simulink model "wrench_observer_R2016b"  (R2016b)
settings: Solver=VariableStepAuto  StartTime=0.0  StopTime=0.75  RelTol=1e-3
InitFcn:
  | %x_k1 = 0.00001*ones(36,1); % initialisation with initial state uncertainity
  | %P_k1 = 0.00001*ones(36); % initialisation with initial state uncertainity
values from neighbouring files (symbols this model uses):
  a_noise = 0    [parameter.m]
  alpha1 = pi/2    (= 1.57079632679)    [parameter.m]
  alpha2 = 0    [parameter.m]
  alpha3 = 0    [parameter.m]
  angular_noise = 0    [parameter.m]
  g = 9.81    [parameter.m]
  K_f_comm = 1    [parameter.m]
  K_I = [500*eye(3), zeros(3), zeros(3) ... (first row only)    [parameter.m]
  K_tau_comm = 1    [parameter.m]
  K_tau_man_comm = 1    [parameter.m]
  m = 3.9    [parameter.m]
  m_l1 = 0.3    [parameter.m]
  m_l2 = 0.35    [parameter.m]
  m_l3 = 0.35    [parameter.m]
  N_m = 1*diag([(p_noise/(3*noise_factor))^2 (p_noise/(3*noise_factor))^2 (p_noise/(3*noise_factor))^2 (a_noise/(3*noise_factor))^2 (a_noise/(3*noise_factor))^2 (a_noise/(3*noise_factor))^2 (angular_noise/(3*noise_factor))^2 (angular_noise/(3*noise_factor))^2 (angular_noise/(3*noise_factor))^2 (omega_noise/(3*noise_factor))^2 (omega_noise/(3*noise_factor))^2 (omega_noise/(3*noise_factor))^2 (theta_noise/( ...(+272 chars)    [parameter.m]
  N_p = diag(noise_factor_EKF)    [parameter.m]
  omega_dot_noise = 0    [parameter.m]
  omega_noise = 0    [parameter.m]
  p_L1_l1 = [p_L1_x_l1 p_L1_y_l1 p_L1_z_l1]'    [parameter.m]
  p_L2_l2 = [p_L2_x_l2 p_L2_y_l2 p_L2_z_l2]'    [parameter.m]
  p_L3_l3 = [p_L3_x_l3 p_L3_y_l3 p_L3_z_l3]'    [parameter.m]
  p_noise = 0    [parameter.m]
  R_B_L0 = [1 0 0;0 1 0; 0 0 1]    [parameter.m]
  T_delay = 0    [parameter.m]
  T_dis = 0.01    [parameter.m]
  theta_dot_dot_noise = 0    [parameter.m]
  theta_dot_noise = 0    [parameter.m]
  theta_noise = 0    [parameter.m]
  Ts = 1/250    (= 0.004)    [parameter.m]
  v_noise = 0    [parameter.m]
libraries: simulink x9, dspstat3 x2, dspinverses x1
(part 4 of 5)

== matlab function wrench_observer_R2016b/Subsystem/MATLAB Function ==
  data: theta input; J_transpose output
function J_transpose = fcn(theta)
theta1 = theta(1);
theta2 = theta(2);
theta3 = theta(3);
% J = [ -cos(theta1)*((3*sin(theta2 + theta3))/10 + (3*sin(theta2))/10), -(3*sin(theta2 + theta3)*cos(theta1))/10,0;
% -sin(theta1)*((3*sin(theta2 + theta3))/10 + (3*sin(theta2))/10), -(3*sin(theta2 + theta3)*sin(theta1))/10,0;
% (3*cos(theta2 + theta3))/10 + (3*cos(theta2))/10,(3*cos(theta2 + theta3))/10,0;
% sin(theta1),sin(theta1),sin(theta1);
% -cos(theta1), -cos(theta1), -cos(theta1);
% 0,0,0];
J = [ -(3*cos(theta2 + theta3)*sin(theta1))/10, -cos(theta1)*((3*sin(theta2 + theta3))/10 - 1/10), -(3*cos(theta1)*(sin(theta2 + theta3) - sin(theta2)))/10;
      (3*cos(theta2 + theta3)*cos(theta1))/10, -sin(theta1)*((3*sin(theta2 + theta3))/10 - 1/10), -(3*sin(theta1)*(sin(theta2 + theta3) - sin(theta2)))/10;
      0, (3*cos(theta2 + theta3))/10, (3*cos(theta2 + theta3))/10 - (3*cos(theta2))/10;
      0, sin(theta1),sin(theta1);
      0,-cos(theta1), -cos(theta1);
      1, 0,0];

J_transpose = J';

== matlab function wrench_observer_R2016b/Wrench Observer EKF/MATLAB Function3 ==
  data: C output
function C = fcn()
C = [ 	1, 	0, 	0, 	0, 	0, 	0, 	0, 	0, 	0, 	0, 	0, 	0, 	0, 	0, 	0, 	0, 	0, 	0, 	0, 	0, 	0, 	0, 	0, 	0, 	0, 	0, 	0, 	0, 	0, 	0, 	0, 	0, 	0, 	0, 	0, 	0; 
		0, 	1, 	0, 	0, 	0, 	0, 	0, 	0, 	0, 	0, 	0, 	0, 	0, 	0, 	0, 	0, 	0, 	0, 	0, 	0, 	0, 	0, 	0, 	0, 	0, 	0, 	0, 	0, 	0, 	0, 	0, 	0, 	0, 	0, 	0, 	0; 
		0, 	0, 	1, 	0, 	0, 	0, 	0, 	0, 	0, 	0, 	0, 	0, 	0, 	0, 	0, 	0, 	0, 	0, 	0, 	0, 	0, 	0, 	0, 	0, 	0, 	0, 	0, 	0, 	0, 	0, 	0, 	0, 	0, 	0, 	0, 	0; 
		0, 	0, 	0, 	0, 	0, 	0, 	3783/392000000000 - (3^(1/2)*((3*3^(1/2))/20 - 1/10))/9800000 - (3*3^(1/2))/7000000000, 	- (9*3^(1/2))/28000000000 - (3^(1/2)*((3*3^(1/2))/20 - 1/10))/9800000 - 52641/784000000000, 	- (3*3^(1/2))/28000000000 - (3^(1/2)*((3*3^(1/2))/20 - 1/10))/4900000 - 53013/784000000000, 	- (3*3^(1/2))/2800000 - 3/9800000, 	381/7840000, 	- (3*3^(1/2))/2800000 - (3^(1/2)*((3*3^(1/2))/20 - 1/10))/1960 - 237/156800000, 	(35937*3^(1/2))/7840000000000 + 1/490000000, 	(35397*3^(1/2))/7840000000000 + 9/28000000000, 	(177*3^(1/2))/392000000000 + 3/17500000000, 	- (3*3^(1/2)*((3*3^(1/2))/20 - 1/10))/1960 - 27/196000, 	-687/1600000, 	-23643/156800000, 	10/49, 	0, 	0, 	10/49, 	0, 	0, 	0, 	0, 	0, 	0, 	0, 	0, 	0, 	0, 	0, 	0, 	0, 	0; 
		0, 	0, 	0, 	0, 	0, 	0, 	- (243969*3^(1/2))/3920000000000 - 26389/245000000000, 	(26073*3^(1/2))/1960000000000 - 991/61250000000, 	- (179727*3^(1/2))/3920000000000 - 110003/980000000000, 	-381/784000, 	- (303*3^(1/2))/56000000 - 303/196000000, 	(56073*3^(1/2))/784000000 - 10303/196000000, 	- (3^(1/2)*((3*3^(1/2))/20 - 1/10))/49000000 - 60189/7840000000000, 	(249*3^(1/2))/392000000000 - 192873/7840000000000, 	- (3561*3^(1/2))/784000000000 - 990219/39200000000000, 	(3*3^(1/2))/39200 - 3/9800, 	- (35979*3^(1/2))/78400000 - 3/9800, 	- (23979*3^(1/2))/156800000 - 3/112000, 	0, 	10/49, 	0, 	0, 	10/49, 	0, 	0, 	0, 	0, 	0, 	0, 	0, 	0, 	0, 	0, 	0, 	0, 	0; 
		0, 	0, 	0, 	0, 	0, 	0, 	(39969*3^(1/2))/392000000000 + (3^(1/2)*((3*3^(1/2))/20 - 1/10))/9800000 + 5337/196000000000, 	(3^(1/2)*((3*3^(1/2))/20 - 1/10))/9800000 - (24273*3^(1/2))/392000000000 + 1429/14000000000, 	(561*3^(1/2))/56000000000 + 5331/196000000000, 	(3*3^(1/2))/28000 + (3^(1/2)*((3*3^(1/2))/20 - 1/10))/1960 + 237/1568000, 	5003/9800000 - (60231*3^(1/2))/78400000, 	0, 	(183*3^(1/2))/78400000000 + (3^(1/2)*((3*3^(1/2))/20 - 1/10))/9800000 - 611/784000000000, 	24147/784000000000 - (14871*3^(1/2))/3920000000000, 	17601/980000000000 - (24021*3^(1/2))/7840000000000, 	(3^(1/2)*((3*3^(1/2))/20 - 1/10))/1960 - (9*3^(1/2))/19600 + 1/1960, 	(2379*3^(1/2))/7840000 + 9/112000, 	(4779*3^(1/2))/15680000 + 9/224000, 	0, 	0, 	10/49, 	0, 	0, 	10/49, 	0, 	0, 	0, 	0, 	0, 	0, 	0, 	0, 	0, 	0, 	0, 	0; 
		0, 	0, 	0, 	0, 	0, 	0, 	1, 	0, 	0, 	0, 	0, 	0, 	0, 	0, 	0, 	0, 	0, 	0, 	0, 	0, 	0, 	0, 	0, 	0, 	0, 	0, 	0, 	0, 	0, 	0, 	0, 	0, 	0, 	0, 	0, 	0; 
		0, 	0, 	0, 	0, 	0, 	0, 	0, 	1, 	0, 	0, 	0, 	0, 	0, 	0, 	0, 	0, 	0, 	0, 	0, 	0, 	0, 	0, 	0, 	0, 	0, 	0, 	0, 	0, 	0, 	0, 	0, 	0, 	0, 	0, 	0, 	0; 
		0, 	0, 	0, 	0, 	0, 	0, 	0, 	0, 	1, 	0, 	0, 	0, 	0, 	0, 	0, 	0, 	0, 	0, 	0, 	0, 	0, 	0, 	0, 	0, 	0, 	0, 	0, 	0, 	0, 	0, 	0, 	0, 	0, 	0, 	0, 	0; 
		0, 	0, 	0, 	0, 	0, 	0, 	0, 	0, 	0, 	1, 	0, 	0, 	0, 	0, 	0, 	0, 	0, 	0, 	0, 	0, 	0, 	0, 	0, 	0, 	0, 	0, 	0, 	0, 	0, 	0, 	0, 	0, 	0, 	0, 	0, 	0; 
		0, 	0, 	0, 	0, 	0, 	0, 	0, 	0, 	0, 	0, 	1, 	0, 	0, 	0, 	0, 	0, 	0, 	0, 	0, 	0, 	0, 	0, 	0, 	0, 	0, 	0, 	0, 	0, 	0, 	0, 	0, 	0, 	0, 	0, 	0, 	0; 
		0, 	0, 	0, 	0, 	0, 	0, 	0, 	0, 	0, 	0, 	0, 	1, 	0, 	0, 	0, 	0, 	0, 	0, 	0, 	0, 	0, 	0, 	0, 	0, 	0, 	0, 	0, 	0, 	0, 	0, 	0, 	0, 	0, 	0, 	0, 	0; 
		0, 	0, 	0, 	0, 	0, 	0, 	0, 	0, 	0, 	0, 	0, 	0, 	1, 	0, 	0, 	0, 	0, 	0, 	0, 	0, 	0, 	0, 	0, 	0, 	0, 	0, 	0, 	0, 	0, 	0, 	0, 	0, 	0, 	0, 	0, 	0; 
		0, 	0, 	0, 	0, 	0, 	0, 	0, 	0, 	0, 	0, 	0, 	0, 	0, 	1, 	0, 	0, 	0, 	0, 	0, 	0, 	0, 	0, 	0, 	0, 	0, 	0, 	0, 	0, 	0, 	0, 	0, 	0, 	0, 	0, 	0, 	0; 
		0, 	0, 	0, 	0, 	0, 	0, 	0, 	0, 	0, 	0, 	0, 	0, 	0, 	0, 	1, 	0, 	0, 	0, 	0, 	0, 	0, 	0, 	0, 	0, 	0, 	0, 	0, 	0, 	0, 	0, 	0, 	0, 	0, 	0, 	0, 	0; 
		0, 	0, 	0, 	((3^(1/2)*((3*3^(1/2))/20 - 1/10))/400 + 27/40000)/(100*((3*3^(1/2))/100000000 - 31/400000000)) + 28569/(6400000000*((3*3^(1/2))/100000000 - 31/400000000)), 	((3*3^(1/2))/8000 + 1/1000)/(100*((3*3^(1/2))/100000000 - 31/400000000)) - ((21*3^(1/2))/16000000 + 3/2000)/(200*((3*3^(1/2))/100000000 - 31/400000000)) + ((23979*3^(1/2))/32000000 + 21/160000)/(200*((3*3^(1/2))/100000000 - 31/400000000)), 	((21*3^(1/2))/1600000 - 63/160000)/(200*((3*3^(1/2))/100000000 - 31/400000000)) - ((4779*3^(1/2))/3200000 + 63/320000)/(200*((3*3^(1/2))/100000000 - 31/400000000)) - ((3^(1/2)*((3*3^(1/2))/20 - 1/10))/400 - (9*3^(1/2))/4000 + 1/400)/(100*((3*3^(1/2))/100000000 - 31/400000000)), 	((5121*3^(1/2)*((3*3^(1/2))/20 - 1/10))/40000000000000 - (4876773983*3^(1/2))/32000000000000000 + 111056949/800000000000000)/(100*((3*3^(1/2))/100000000 - 31/400000000)) - ((9397082859*3^(1/2))/64000000000000000 + (21*3^(1/2)*((3*3^(1/2))/20 - 1/10))/160000000000 + 346647/20000000000000)/(200*((3*3^(1/2))/100000000 - 31/400000000)) - ((1183480443*3^(1/2))/80000000000000000 + (21*3^(1/2)*((3*3^(1/2))/20 - 1/10))/3200000000000 - 16010785891/800000000000000)/(10*((3*3^(1/2))/100000000 - 31/400000000)) + ((1665944541*3^(1/2))/32000000000000000 + (3831*3^(1/2)*((3*3^(1/2))/20 - 1/10))/200000000000000 - 160128933757/8000000000000000)/(5*((3*3^(1/2))/100000000 - 31/400000000)) + ((377787*3^(1/2))/200000000000000 - 27893859/80000000000000)/(200*((3*3^(1/2))/100000000 - 31/400000000)) + ((5185251*3^(1/2))/16000000000000000 + 31944083711/1600000000000000)/(10*((3*3^(1/2))/100000000 - 31/400000000)) - (((21*3^(1/2))/20000000 - 217/80000000)*((5185251*3^(1/2))/16000000000000000 + 31944083711/1600000000000000))/(200*((3*3^(1/2))/100000000 - 31/400000000)^2) + (((21*3^(1/2))/20000000 - 217/80000000)*((1183480443*3^(1/2))/80000000000000000 + (21*3^(1/2)*((3*3^(1/2))/20 - 1/10))/3200000000000 - 16010785891/800000000000000))/(200*((3*3^(1/2))/100000000 - 31/400000000)^2) - (((21*3^(1/2))/20000000 - 217/80000000)*((1665944541*3^(1/2))/32000000000000000 + (3831*3^(1/2)*((3*3^(1/2))/20 - 1/10))/200000000000000 - 160128933757/8000000000000000))/(100*((3*3^(1/2))/100000000 - 31/400000000)^2), 	((1665944541*3^(1/2))/32000000000000000 + (3831*3^(1/2)*((3*3^(1/2))/20 - 1/10))/200000000000000 - 160128933757/8000000000000000)/(5*((3*3^(1/2))/100000000 - 31/400000000)) - ((3795389037*3^(1/2))/12800000000000000 + (21*3^(1/2)*((3*3^(1/2))/20 - 1/10))/320000000000 - 27840879/160000000000000)/(200*((3*3^(1/2))/100000000 - 31/400000000)) - ((1183480443*3^(1/2))/80000000000000000 + (21*3^(1/2)*((3*3^(1/2))/20 - 1/10))/3200000000000 - 16010785891/800000000000000)/(10*((3*3^(1/2))/100000000 - 31/400000000)) - ((2482807*3^(1/2)*((3*3^(1/2))/20 - 1/10))/5000000000000 - (11772968963*3^(1/2))/32000000000000000 + 61404471/200000000000000)/(100*((3*3^(1/2))/100000000 - 31/400000000)) + ((3210399*3^(1/2))/800000000000000 - (3*3^(1/2)*((3*3^(1/2))/20 - 1/10))/2000000000 + 4331121/160000000000000)/(200*((3*3^(1/2))/100000000 - 31/400000000)) + ((5185251*3^(1/2))/16000000000000000 + 31944083711/1600000000000000)/(10*((3*3^(1/2))/100000000 - 31/400000000)) + (((3*3^(1/2))/4000000 - 31/16000000)*((1183480443*3^(1/2))/80000000000000000 + (21*3^(1/2)*((3*3^(1/2))/20 - 1/10))/3200000000000 - 16010785891/800000000000000))/(200*((3*3^(1/2))/100000000 - 31/400000000)^2) - (((3*3^(1/2))/4000000 - 31/16000000)*((1665944541*3^(1/2))/32000000000000000 + (3831*3^(1/2)*((3*3^(1/2))/20 - 1/10))/200000000000000 - 160128933757/8000000000000000))/(100*((3*3^(1/2))/100000000 - 31/400000000)^2) - (((3*3^(1/2))/4000000 - 31/16000000)*((5185251*3^(1/2))/16000000000000000 + 31944083711/1600000000000000))/(200*((3*3^(1/2))/100000000 - 31/400000000)^2), 	((114343521*3^(1/2))/1600000000000000 + (9943777*3^(1/2)*((3*3^(1/2))/20 - 1/10))/20000000000000 + 268316551/800000000000000)/(100*((3*3^(1/2))/100000000 - 31/400000000)) + ((3465639*3^(1/2))/1600000000000000 + (3*3^(1/2)*((3*3^(1/2))/20 - 1/10))/2000000000 - 55575441/160000000000000)/(200*((3*3^(1/2))/100000000 - 31/400000000)) + ((2404758213*3^(1/2))/16000000000000000 - (21*3^(1/2)*((3*3^(1/2))/20 - 1/10))/320000000000 + 7131903/64000000000000)/(200*((3*3^(1/2))/100000000 - 31/400000000)) + (((3*3^(1/2))/5000000 - 31/20000000)*((1183480443*3^(1/2))/80000000000000000 + (21*3^(1/2)*((3*3^(1/2))/20 - 1/10))/3200000000000 - 16010785891/800000000000000))/(200*((3*3^(1/2))/100000000 - 31/400000000)^2) - (((3*3^(1/2))/5000000 - 31/20000000)*((1665944541*3^(1/2))/32000000000000000 + (3831*3^(1/2)*((3*3^(1/2))/20 - 1/10))/200000000000000 - 160128933757/8000000000000000))/(100*((3*3^(1/2))/100000000 - 31/400000000)^2) - (((3*3^(1/2))/5000000 - 31/20000000)*((5185251*3^(1/2))/16000000000000000 + 31944083711/1600000000000000))/(200*((3*3^(1/2))/100000000 - 31/400000000)^2), 	- ((62493*3^(1/2))/16000000000 + (249937*3^(1/2)*((3*3^(1/2))/20 - 1/10))/100000000 - 23974611/32000000000)/(100*((3*3^(1/2))/100000000 - 31/400000000)) - 60604689/(6400000000000*((3*3^(1/2))/100000000 - 31/400000000)) - ((207*3^(1/2))/1280000000 + (21*3^(1/2)*((3*3^(1/2))/20 - 1/10))/32000000 + 2114643/32000000000)/(200*((3*3^(1/2))/100000000 - 31/400000000)), 	((2107047*3^(1/2))/320000000000 - 168129/12800000000)/(200*((3*3^(1/2))/100000000 - 31/400000000)) + ((7765251*3^(1/2))/320000000000 + 5703/40000000)/(200*((3*3^(1/2))/100000000 - 31/400000000)) - ((3*3^(1/2)*((3*3^(1/2))/20 - 1/10))/8000000000 - (596441019*3^(1/2))/160000000000 + 204842381/80000000000)/(100*((3*3^(1/2))/100000000 - 31/400000000)), 	((20010287*3^(1/2)*((3*3^(1/2))/20 - 1/10))/8000000000 - (119986137*3^(1/2))/320000000000 + 40005943/160000000000)/(100*((3*3^(1/2))/100000000 - 31/400000000)) - ((1031871*3^(1/2))/1600000000000 - 121359/64000000000)/(200*((3*3^(1/2))/100000000 - 31/400000000)) - ((416349*3^(1/2))/320000000000 - 123711/32000000000)/(200*((3*3^(1/2))/100000000 - 31/400000000)), 	- ((4034511*3^(1/2))/1600000000000000 + (297*3^(1/2)*((3*3^(1/2))/20 - 1/10))/400000000000 + 16684749/16000000000000000)/(200*((3*3^(1/2))/100000000 - 31/400000000)) - ((7589019*3^(1/2))/500000000000000 + (179409213*3^(1/2)*((3*3^(1/2))/20 - 1/10))/400000000000000 - 125998557/8000000000000000)/(100*((3*3^(1/2))/100000000 - 31/400000000)) - ((52161039*3^(1/2))/3200000000000000 + (21*3^(1/2)*((3*3^(1/2))/20 - 1/10))/32000000000000 - 117174411/8000000000000000)/(200*((3*3^(1/2))/100000000 - 31/400000000)), 	((1183480443*3^(1/2))/80000000000000000 + (21*3^(1/2)*((3*3^(1/2))/20 - 1/10))/3200000000000 - 16010785891/800000000000000)/(300*((3*3^(1/2))/100000000 - 31/400000000)) + ((78898791*3^(1/2))/4000000000000000 + (21*3^(1/2)*((3*3^(1/2))/20 - 1/10))/16000000000000 + 2373464247/20000000000000000)/(200*((3*3^(1/2))/100000000 - 31/400000000)) + ((29906877*3^(1/2))/1600000000000000 + (21*3^(1/2)*((3*3^(1/2))/20 - 1/10))/32000000000000 + 5990219349/80000000000000000)/(200*((3*3^(1/2))/100000000 - 31/400000000)) + ((5185251*3^(1/2))/16000000000000000 + 31944083711/1600000000000000)/(300*((3*3^(1/2))/100000000 - 31/400000000)) - ((23697*3^(1/2)*((3*3^(1/2))/20 - 1/10))/32000000000000 - (369986349*3^(1/2))/8000000000000000 + 51614439/8000000000000000)/(100*((3*3^(1/2))/100000000 - 31/400000000)), 	((599887743*3^(1/2))/16000000000000000 - (1779879*3^(1/2)*((3*3^(1/2))/20 - 1/10))/1600000000000000 + 14540151/32000000000000000)/(100*((3*3^(1/2))/100000000 - 31/400000000)) + ((11901*3^(1/2)*((3*3^(1/2))/20 - 1/10))/32000000000000 - (4750881*3^(1/2))/2000000000000000 + 4731132549/80000000000000000)/(200*((3*3^(1/2))/100000000 - 31/400000000)) + ((29900577*3^(1/2))/1600000000000000 + (21*3^(1/2)*((3*3^(1/2))/20 - 1/10))/32000000000000 + 5997450849/80000000000000000)/(200*((3*3^(1/2))/100000000 - 31/400000000)) + (((11*3^(1/2))/200000000 - 3/40000000)*((5185251*3^(1/2))/16000000000000000 + 31944083711/1600000000000000))/(200*((3*3^(1/2))/100000000 - 31/400000000)^2) - (100*((3*3^(1/2))/20000 - 1/20000)*((1183480443*3^(1/2))/80000000000000000 + (21*3^(1/2)*((3*3^(1/2))/20 - 1/10))/3200000000000 - 16010785891/800000000000000))/(3*((3*3^(1/2))/100000000 - 31/400000000)) - (((11*3^(1/2))/200000000 - 3/40000000)*((1183480443*3^(1/2))/80000000000000000 + (21*3^(1/2)*((3*3^(1/2))/20 - 1/10))/3200000000000 - 16010785891/800000000000000))/(200*((3*3^(1/2))/100000000 - 31/400000000)^2) + (((11*3^(1/2))/200000000 - 3/40000000)*((1665944541*3^(1/2))/32000000000000000 + (3831*3^(1/2)*((3*3^(1/2))/20 - 1/10))/200000000000000 - 160128933757/8000000000000000))/(100*((3*3^(1/2))/100000000 - 31/400000000)^2) + (3^(1/2)*((1665944541*3^(1/2))/32000000000000000 + (3831*3^(1/2)*((3*3^(1/2))/20 - 1/10))/200000000000000 - 160128933757/8000000000000000))/(100*((3*3^(1/2))/100000000 - 31/400000000)) + (100*((3*3^(1/2))/20000 + 1/20000)*((5185251*3^(1/2))/16000000000000000 + 31944083711/1600000000000000))/(3*((3*3^(1/2))/100000000 - 31/400000000)), 	- ((891*3^(1/2))/80000000 - 417/40000000)/(100*((3*3^(1/2))/100000000 - 31/400000000)) - ((1192731*3^(1/2))/3200000000 - 1205067/3200000000)/(200*((3*3^(1/2))/100000000 - 31/400000000)) - ((292941*3^(1/2))/800000000 - 589209/1600000000)/(200*((3*3^(1/2))/100000000 - 31/400000000)), 	- (9*3^(1/2))/(400000000*((3*3^(1/2))/100000000 - 31/400000000)) - ((58929*3^(1/2))/160000000 - 601209/1600000000)/(200*((3*3^(1/2))/100000000 - 31/400000000)) - ((307161*3^(1/2))/800000000 - 620169/1600000000)/(100*((3*3^(1/2))/100000000 - 31/400000000)), 	((58929*3^(1/2))/160000000 - 601209/1600000000)/(200*((3*3^(1/2))/100000000 - 31/400000000)) - ((1192731*3^(1/2))/3200000000 - 1205067/3200000000)/(100*((3*3^(1/2))/100000000 - 31/400000000)), 	0, 	0, 	0, 	0, 	0, 	0, 	0, 	0, 	0, 	0, 	0, 	0, 	-1/(100*((3*3^(1/2))/100000000 - 31/400000000)), 	1/(200*((3*3^(1/2))/100000000 - 31/400000000)), 	1/(200*((3*3^(1/2))/100000000 - 31/400000000)), 	-1/(100*((3*3^(1/2))/100000000 - 31/400000000)), 	1/(200*((3*3^(1/2))/100000000 - 31/400000000)), 	1/(200*((3*3^(1/2))/100000000 - 31/400000000)); 
		0, 	0, 	0, 	(821*((3*3^(1/2))/10000 - 1/1000))/(480000*((3*3^(1/2))/100000000 - 31/400000000)) - (2627*((3*3^(1/2))/10000 - 11/20000))/(320000*((3*3^(1/2))/100000000 - 31/400000000)) - ((3^(1/2)*((3*3^(1/2))/20 - 1/10))/400 + 27/40000)/(200*((3*3^(1/2))/100000000 - 31/400000000)), 	- ((3*3^(1/2))/8000 + 1/1000)/(200*((3*3^(1/2))/100000000 - 31/400000000)) - (100*((3*3^(1/2))/10000 - 1/1000)*((21*3^(1/2))/16000000 + 3/2000))/(9*((3*3^(1/2))/100000000 - 31/400000000)) - (100*((3*3^(1/2))/10000 - 11/20000)*((23979*3^(1/2))/32000000 + 21/160000))/(9*((3*3^(1/2))/100000000 - 31/400000000)), 	((3^(1/2)*((3*3^(1/2))/20 - 1/10))/400 - (9*3^(1/2))/4000 + 1/400)/(200*((3*3^(1/2))/100000000 - 31/400000000)) + (100*((3*3^(1/2))/10000 - 1/1000)*((21*3^(1/2))/1600000 - 63/160000))/(9*((3*3^(1/2))/100000000 - 31/400000000)) + (100*((3*3^(1/2))/10000 - 11/20000)*((4779*3^(1/2))/3200000 + 63/320000))/(9*((3*3^(1/2))/100000000 - 31/400000000)), 	(100*((9*3^(1/2))/2000 - 57/8000)*((1183480443*3^(1/2))/80000000000000000 + (21*3^(1/2)*((3*3^(1/2))/20 - 1/10))/3200000000000 - 16010785891/800000000000000))/(9*((3*3^(1/2))/100000000 - 31/400000000)) - ((1665944541*3^(1/2))/32000000000000000 + (3831*3^(1/2)*((3*3^(1/2))/20 - 1/10))/200000000000000 - 160128933757/8000000000000000)/(10*((3*3^(1/2))/100000000 - 31/400000000)) - ((5121*3^(1/2)*((3*3^(1/2))/20 - 1/10))/40000000000000 - (4876773983*3^(1/2))/32000000000000000 + 111056949/800000000000000)/(200*((3*3^(1/2))/100000000 - 31/400000000)) + (100*((3*3^(1/2))/10000 - 11/20000)*((9397082859*3^(1/2))/64000000000000000 + (21*3^(1/2)*((3*3^(1/2))/20 - 1/10))/160000000000 + 346647/20000000000000))/(9*((3*3^(1/2))/100000000 - 31/400000000)) + (((21*3^(1/2))/20000000 - 217/80000000)*((1665944541*3^(1/2))/32000000000000000 + (3831*3^(1/2)*((3*3^(1/2))/20 - 1/10))/200000000000000 - 160128933757/8000000000000000))/(200*((3*3^(1/2))/100000000 - 31/400000000)^2) + (100*((3*3^(1/2))/10000 - 1/1000)*((377787*3^(1/2))/200000000000000 - 27893859/80000000000000))/(9*((3*3^(1/2))/100000000 - 31/400000000)) + (100*((9*3^(1/2))/2000 - 129/8000)*((5185251*3^(1/2))/16000000000000000 + 31944083711/1600000000000000))/(9*((3*3^(1/2))/100000000 - 31/400000000)) - (100*((3*3^(1/2))/10000 - 1/1000)*((21*3^(1/2))/20000000 - 217/80000000)*((5185251*3^(1/2))/16000000000000000 + 31944083711/1600000000000000))/(9*((3*3^(1/2))/100000000 - 31/400000000)^2) - (100*((3*3^(1/2))/10000 - 11/20000)*((21*3^(1/2))/20000000 - 217/80000000)*((1183480443*3^(1/2))/80000000000000000 + (21*3^(1/2)*((3*3^(1/2))/20 - 1/10))/3200000000000 - 16010785891/800000000000000))/(9*((3*3^(1/2))/100000000 - 31/400000000)^2), 	((2482807*3^(1/2)*((3*3^(1/2))/20 - 1/10))/5000000000000 - (11772968963*3^(1/2))/32000000000000000 + 61404471/200000000000000)/(200*((3*3^(1/2))/100000000 - 31/400000000)) - ((1665944541*3^(1/2))/32000000000000000 + (3831*3^(1/2)*((3*3^(1/2))/20 - 1/10))/200000000000000 - 160128933757/8000000000000000)/(10*((3*3^(1/2))/100000000 - 31/400000000)) + (100*((3*3^(1/2))/2000 + 1/1600)*((1183480443*3^(1/2))/80000000000000000 + (21*3^(1/2)*((3*3^(1/2))/20 - 1/10))/3200000000000 - 16010785891/800000000000000))/(9*((3*3^(1/2))/100000000 - 31/400000000)) + (100*((3*3^(1/2))/10000 - 11/20000)*((3795389037*3^(1/2))/12800000000000000 + (21*3^(1/2)*((3*3^(1/2))/20 - 1/10))/320000000000 - 27840879/160000000000000))/(9*((3*3^(1/2))/100000000 - 31/400000000)) + (((3*3^(1/2))/4000000 - 31/16000000)*((1665944541*3^(1/2))/32000000000000000 + (3831*3^(1/2)*((3*3^(1/2))/20 - 1/10))/200000000000000 - 160128933757/8000000000000000))/(200*((3*3^(1/2))/100000000 - 31/400000000)^2) + (100*((3*3^(1/2))/10000 - 1/1000)*((3210399*3^(1/2))/800000000000000 - (3*3^(1/2)*((3*3^(1/2))/20 - 1/10))/2000000000 + 4331121/160000000000000))/(9*((3*3^(1/2))/100000000 - 31/400000000)) + (100*((3*3^(1/2))/2000 - 67/8000)*((5185251*3^(1/2))/16000000000000000 + 31944083711/1600000000000000))/(9*((3*3^(1/2))/100000000 - 31/400000000)) - (100*((3*3^(1/2))/10000 - 1/1000)*((3*3^(1/2))/4000000 - 31/16000000)*((5185251*3^(1/2))/16000000000000000 + 31944083711/1600000000000000))/(9*((3*3^(1/2))/100000000 - 31/400000000)^2) - (100*((3*3^(1/2))/10000 - 11/20000)*((3*3^(1/2))/4000000 - 31/16000000)*((1183480443*3^(1/2))/80000000000000000 + (21*3^(1/2)*((3*3^(1/2))/20 - 1/10))/3200000000000 - 16010785891/800000000000000))/(9*((3*3^(1/2))/100000000 - 31/400000000)^2), 	(100*((3*3^(1/2))/500 - 31/2000)*((1183480443*3^(1/2))/80000000000000000 + (21*3^(1/2)*((3*3^(1/2))/20 - 1/10))/3200000000000 - 16010785891/800000000000000))/(9*((3*3^(1/2))/100000000 - 31/400000000)) - ((114343521*3^(1/2))/1600000000000000 + (9943777*3^(1/2)*((3*3^(1/2))/20 - 1/10))/20000000000000 + 268316551/800000000000000)/(200*((3*3^(1/2))/100000000 - 31/400000000)) + (100*((3*3^(1/2))/10000 - 1/1000)*((3465639*3^(1/2))/1600000000000000 + (3*3^(1/2)*((3*3^(1/2))/20 - 1/10))/2000000000 - 55575441/160000000000000))/(9*((3*3^(1/2))/100000000 - 31/400000000)) - (100*((3*3^(1/2))/10000 - 11/20000)*((2404758213*3^(1/2))/16000000000000000 - (21*3^(1/2)*((3*3^(1/2))/20 - 1/10))/320000000000 + 7131903/64000000000000))/(9*((3*3^(1/2))/100000000 - 31/400000000)) + (((3*3^(1/2))/5000000 - 31/20000000)*((1665944541*3^(1/2))/32000000000000000 + (3831*3^(1/2)*((3*3^(1/2))/20 - 1/10))/200000000000000 - 160128933757/8000000000000000))/(200*((3*3^(1/2))/100000000 - 31/400000000)^2) + (100*((3*3^(1/2))/500 - 31/2000)*((5185251*3^(1/2))/16000000000000000 + 31944083711/1600000000000000))/(9*((3*3^(1/2))/100000000 - 31/400000000)) - (100*((3*3^(1/2))/10000 - 1/1000)*((3*3^(1/2))/5000000 - 31/20000000)*((5185251*3^(1/2))/16000000000000000 + 31944083711/1600000000000000))/(9*((3*3^(1/2))/100000000 - 31/400000000)^2) - (100*((3*3^(1/2))/10000 - 11/20000)*((3*3^(1/2))/5000000 - 31/20000000)*((1183480443*3^(1/2))/80000000000000000 + (21*3^(1/2)*((3*3^(1/2))/20 - 1/10))/3200000000000 - 16010785891/800000000000000))/(9*((3*3^(1/2))/100000000 - 31/400000000)^2), 	((62493*3^(1/2))/16000000000 + (249937*3^(1/2)*((3*3^(1/2))/20 - 1/10))/100000000 - 23974611/32000000000)/(200*((3*3^(1/2))/100000000 - 31/400000000)) - (20201563*((3*3^(1/2))/10000 - 1/1000))/(960000000*((3*3^(1/2))/100000000 - 31/400000000)) + (100*((3*3^(1/2))/10000 - 11/20000)*((207*3^(1/2))/1280000000 + (21*3^(1/2)*((3*3^(1/2))/20 - 1/10))/32000000 + 2114643/32000000000))/(9*((3*3^(1/2))/100000000 - 31/400000000)), 	((3*3^(1/2)*((3*3^(1/2))/20 - 1/10))/8000000000 - (596441019*3^(1/2))/160000000000 + 204842381/80000000000)/(200*((3*3^(1/2))/100000000 - 31/400000000)) - (100*((3*3^(1/2))/10000 - 11/20000)*((2107047*3^(1/2))/320000000000 - 168129/12800000000))/(9*((3*3^(1/2))/100000000 - 31/400000000)) + (100*((3*3^(1/2))/10000 - 1/1000)*((7765251*3^(1/2))/320000000000 + 5703/40000000))/(9*((3*3^(1/2))/100000000 - 31/400000000)), 	(100*((3*3^(1/2))/10000 - 11/20000)*((1031871*3^(1/2))/1600000000000 - 121359/64000000000))/(9*((3*3^(1/2))/100000000 - 31/400000000)) - (100*((416349*3^(1/2))/320000000000 - 123711/32000000000)*((3*3^(1/2))/10000 - 1/1000))/(9*((3*3^(1/2))/100000000 - 31/400000000)) - ((20010287*3^(1/2)*((3*3^(1/2))/20 - 1/10))/8000000000 - (119986137*3^(1/2))/320000000000 + 40005943/160000000000)/(200*((3*3^(1/2))/100000000 - 31/400000000)), 	((7589019*3^(1/2))/500000000000000 + (179409213*3^(1/2)*((3*3^(1/2))/20 - 1/10))/400000000000000 - 125998557/8000000000000000)/(200*((3*3^(1/2))/100000000 - 31/400000000)) - (100*((3*3^(1/2))/10000 - 1/1000)*((4034511*3^(1/2))/1600000000000000 + (297*3^(1/2)*((3*3^(1/2))/20 - 1/10))/400000000000 + 16684749/16000000000000000))/(9*((3*3^(1/2))/100000000 - 31/400000000)) + (100*((3*3^(1/2))/10000 - 11/20000)*((52161039*3^(1/2))/3200000000000000 + (21*3^(1/2)*((3*3^(1/2))/20 - 1/10))/32000000000000 - 117174411/8000000000000000))/(9*((3*3^(1/2))/100000000 - 31/400000000)), 	((23697*3^(1/2)*((3*3^(1/2))/20 - 1/10))/32000000000000 - (369986349*3^(1/2))/8000000000000000 + 51614439/8000000000000000)/(200*((3*3^(1/2))/100000000 - 31/400000000)) - ((5185251*3^(1/2))/16000000000000000 + 31944083711/1600000000000000)/(300*((3*3^(1/2))/100000000 - 31/400000000)) - ((1665944541*3^(1/2))/32000000000000000 + (3831*3^(1/2)*((3*3^(1/2))/20 - 1/10))/200000000000000 - 160128933757/8000000000000000)/(300*((3*3^(1/2))/100000000 - 31/400000000)) + (100*((3*3^(1/2))/10000 - 1/1000)*((78898791*3^(1/2))/4000000000000000 + (21*3^(1/2)*((3*3^(1/2))/20 - 1/10))/16000000000000 + 2373464247/20000000000000000))/(9*((3*3^(1/2))/100000000 - 31/400000000)) - (100*((3*3^(1/2))/10000 - 11/20000)*((29906877*3^(1/2))/1600000000000000 + (21*3^(1/2)*((3*3^(1/2))/20 - 1/10))/32000000000000 + 5990219349/80000000000000000))/(9*((3*3^(1/2))/100000000 - 31/400000000)), 	(100*((9*3^(1/2))/20000 - 3/20000)*((1183480443*3^(1/2))/80000000000000000 + (21*3^(1/2)*((3*3^(1/2))/20 - 1/10))/3200000000000 - 16010785891/800000000000000))/(9*((3*3^(1/2))/100000000 - 31/400000000)) - ((5185251*3^(1/2))/16000000000000000 + 31944083711/1600000000000000)/(300*((3*3^(1/2))/100000000 - 31/400000000)) - ((599887743*3^(1/2))/16000000000000000 - (1779879*3^(1/2)*((3*3^(1/2))/20 - 1/10))/1600000000000000 + 14540151/32000000000000000)/(200*((3*3^(1/2))/100000000 - 31/400000000)) + (100*((3*3^(1/2))/10000 - 1/1000)*((11901*3^(1/2)*((3*3^(1/2))/20 - 1/10))/32000000000000 - (4750881*3^(1/2))/2000000000000000 + 4731132549/80000000000000000))/(9*((3*3^(1/2))/100000000 - 31/400000000)) - (100*((3*3^(1/2))/10000 - 11/20000)*((29900577*3^(1/2))/1600000000000000 + (21*3^(1/2)*((3*3^(1/2))/20 - 1/10))/32000000000000 + 5997450849/80000000000000000))/(9*((3*3^(1/2))/100000000 - 31/400000000)) - (100*((3*3^(1/2))/20000 + 1/20000)*((1665944541*3^(1/2))/32000000000000000 + (3831*3^(1/2)*((3*3^(1/2))/20 - 1/10))/200000000000000 - 160128933757/8000000000000000))/(3*((3*3^(1/2))/100000000 - 31/400000000)) - (((11*3^(1/2))/200000000 - 3/40000000)*((1665944541*3^(1/2))/32000000000000000 + (3831*3^(1/2)*((3*3^(1/2))/20 - 1/10))/200000000000000 - 160128933757/8000000000000000))/(200*((3*3^(1/2))/100000000 - 31/400000000)^2) + (100*((3*3^(1/2))/10000 - 1/1000)*((11*3^(1/2))/200000000 - 3/40000000)*((5185251*3^(1/2))/16000000000000000 + 31944083711/1600000000000000))/(9*((3*3^(1/2))/100000000 - 31/400000000)^2) + (100*((3*3^(1/2))/10000 - 11/20000)*((11*3^(1/2))/200000000 - 3/40000000)*((1183480443*3^(1/2))/80000000000000000 + (21*3^(1/2)*((3*3^(1/2))/20 - 1/10))/3200000000000 - 16010785891/800000000000000))/(9*((3*3^(1/2))/100000000 - 31/400000000)^2), 	((891*3^(1/2))/80000000 - 417/40000000)/(200*((3*3^(1/2))/100000000 - 31/400000000)) + (100*((3*3^(1/2))/10000 - 11/20000)*((1192731*3^(1/2))/3200000000 - 1205067/3200000000))/(9*((3*3^(1/2))/100000000 - 31/400000000)) - (100*((3*3^(1/2))/10000 - 1/1000)*((292941*3^(1/2))/800000000 - 589209/1600000000))/(9*((3*3^(1/2))/100000000 - 31/400000000)), 	((307161*3^(1/2))/800000000 - 620169/1600000000)/(200*((3*3^(1/2))/100000000 - 31/400000000)) - (3^(1/2)*((3*3^(1/2))/10000 - 1/1000))/(20000*((3*3^(1/2))/100000000 - 31/400000000)) + (100*((3*3^(1/2))/10000 - 11/20000)*((58929*3^(1/2))/160000000 - 601209/1600000000))/(9*((3*3^(1/2))/100000000 - 31/400000000)), 	((1192731*3^(1/2))/3200000000 - 1205067/3200000000)/(200*((3*3^(1/2))/100000000 - 31/400000000)) + (100*((3*3^(1/2))/10000 - 1/1000)*((58929*3^(1/2))/160000000 - 601209/1600000000))/(9*((3*3^(1/2))/100000000 - 31/400000000)), 	0, 	0, 	0, 	0, 	0, 	0, 	0, 	0, 	0, 	0, 	0, 	0, 	1/(200*((3*3^(1/2))/100000000 - 31/400000000)), 	(100*((3*3^(1/2))/10000 - 1/1000))/(9*((3*3^(1/2))/100000000 - 31/400000000)), 	-(100*((3*3^(1/2))/10000 - 11/20000))/(9*((3*3^(1/2))/100000000 - 31/400000000)), 	1/(200*((3*3^(1/2))/100000000 - 31/400000000)), 	(100*((3*3^(1/2))/10000 - 1/1000))/(9*((3*3^(1/2))/100000000 - 31/400000000)), 	-(100*((3*3^(1/2))/10000 - 11/20000))/(9*((3*3^(1/2))/100000000 - 31/400000000)); 
		0, 	0, 	0, 	(2627*((27009*3^(1/2))/1000000000 - 3489/50000000))/(1600000*((9*3^(1/2))/50000000000000 - 93/200000000000000)) - ((3^(1/2)*((3*3^(1/2))/20 - 1/10))/400 + 27/40000)/(200*((3*3^(1/2))/100000000 - 31/400000000)) - (821*((3*3^(1/2))/10000 - 11/20000))/(480000*((3*3^(1/2))/100000000 - 31/400000000)), 	(20*((23979*3^(1/2))/32000000 + 21/160000)*((27009*3^(1/2))/1000000000 - 3489/50000000))/(9*((9*3^(1/2))/50000000000000 - 93/200000000000000)) - ((3*3^(1/2))/8000 + 1/1000)/(200*((3*3^(1/2))/100000000 - 31/400000000)) + (100*((3*3^(1/2))/10000 - 11/20000)*((21*3^(1/2))/16000000 + 3/2000))/(9*((3*3^(1/2))/100000000 - 31/400000000)), 	((3^(1/2)*((3*3^(1/2))/20 - 1/10))/400 - (9*3^(1/2))/4000 + 1/400)/(200*((3*3^(1/2))/100000000 - 31/400000000)) - (20*((4779*3^(1/2))/3200000 + 63/320000)*((27009*3^(1/2))/1000000000 - 3489/50000000))/(9*((9*3^(1/2))/50000000000000 - 93/200000000000000)) - (100*((3*3^(1/2))/10000 - 11/20000)*((21*3^(1/2))/1600000 - 63/160000))/(9*((3*3^(1/2))/100000000 - 31/400000000)), 	(((21*3^(1/2))/20000000 - 217/80000000)*((1665944541*3^(1/2))/32000000000000000 + (3831*3^(1/2)*((3*3^(1/2))/20 - 1/10))/200000000000000 - 160128933757/8000000000000000))/(200*((3*3^(1/2))/100000000 - 31/400000000)^2) - ((1665944541*3^(1/2))/32000000000000000 + (3831*3^(1/2)*((3*3^(1/2))/20 - 1/10))/200000000000000 - 160128933757/8000000000000000)/(10*((3*3^(1/2))/100000000 - 31/400000000)) - (20*((27009*3^(1/2))/1000000000 - 3489/50000000)*((9397082859*3^(1/2))/64000000000000000 + (21*3^(1/2)*((3*3^(1/2))/20 - 1/10))/160000000000 + 346647/20000000000000))/(9*((9*3^(1/2))/50000000000000 - 93/200000000000000)) - ((5121*3^(1/2)*((3*3^(1/2))/20 - 1/10))/40000000000000 - (4876773983*3^(1/2))/32000000000000000 + 111056949/800000000000000)/(200*((3*3^(1/2))/100000000 - 31/400000000)) - (100*((3*3^(1/2))/10000 - 11/20000)*((377787*3^(1/2))/200000000000000 - 27893859/80000000000000))/(9*((3*3^(1/2))/100000000 - 31/400000000)) - (20*((37809*3^(1/2))/40000000 - 1953627/800000000)*((1183480443*3^(1/2))/80000000000000000 + (21*3^(1/2)*((3*3^(1/2))/20 - 1/10))/3200000000000 - 16010785891/800000000000000))/(9*((9*3^(1/2))/50000000000000 - 93/200000000000000)) - (100*((9*3^(1/2))/2000 - 57/8000)*((5185251*3^(1/2))/16000000000000000 + 31944083711/1600000000000000))/(9*((3*3^(1/2))/100000000 - 31/400000000)) + (100*((3*3^(1/2))/10000 - 11/20000)*((21*3^(1/2))/20000000 - 217/80000000)*((5185251*3^(1/2))/16000000000000000 + 31944083711/1600000000000000))/(9*((3*3^(1/2))/100000000 - 31/400000000)^2) + (20*((27009*3^(1/2))/1000000000 - 3489/50000000)*((81*3^(1/2))/10000000000000 - 837/40000000000000)*((1183480443*3^(1/2))/80000000000000000 + (21*3^(1/2)*((3*3^(1/2))/20 - 1/10))/3200000000000 - 16010785891/800000000000000))/(9*((9*3^(1/2))/50000000000000 - 93/200000000000000)^2), 	((2482807*3^(1/2)*((3*3^(1/2))/20 - 1/10))/5000000000000 - (11772968963*3^(1/2))/32000000000000000 + 61404471/200000000000000)/(200*((3*3^(1/2))/100000000 - 31/400000000)) - ((1665944541*3^(1/2))/32000000000000000 + (3831*3^(1/2)*((3*3^(1/2))/20 - 1/10))/200000000000000 - 160128933757/8000000000000000)/(10*((3*3^(1/2))/100000000 - 31/400000000)) - (20*((27009*3^(1/2))/1000000000 - 3489/50000000)*((3795389037*3^(1/2))/12800000000000000 + (21*3^(1/2)*((3*3^(1/2))/20 - 1/10))/320000000000 - 27840879/160000000000000))/(9*((9*3^(1/2))/50000000000000 - 93/200000000000000)) + (((3*3^(1/2))/4000000 - 31/16000000)*((1665944541*3^(1/2))/32000000000000000 + (3831*3^(1/2)*((3*3^(1/2))/20 - 1/10))/200000000000000 - 160128933757/8000000000000000))/(200*((3*3^(1/2))/100000000 - 31/400000000)^2) - (20*((135063*3^(1/2))/200000000 - 1395921/800000000)*((1183480443*3^(1/2))/80000000000000000 + (21*3^(1/2)*((3*3^(1/2))/20 - 1/10))/3200000000000 - 16010785891/800000000000000))/(9*((9*3^(1/2))/50000000000000 - 93/200000000000000)) - (100*((3*3^(1/2))/10000 - 11/20000)*((3210399*3^(1/2))/800000000000000 - (3*3^(1/2)*((3*3^(1/2))/20 - 1/10))/2000000000 + 4331121/160000000000000))/(9*((3*3^(1/2))/100000000 - 31/400000000)) - (100*((3*3^(1/2))/2000 + 1/1600)*((5185251*3^(1/2))/16000000000000000 + 31944083711/1600000000000000))/(9*((3*3^(1/2))/100000000 - 31/400000000)) + (100*((3*3^(1/2))/10000 - 11/20000)*((3*3^(1/2))/4000000 - 31/16000000)*((5185251*3^(1/2))/16000000000000000 + 31944083711/1600000000000000))/(9*((3*3^(1/2))/100000000 - 31/400000000)^2) + (20*((27009*3^(1/2))/1000000000 - 3489/50000000)*((99*3^(1/2))/10000000000000 - 1023/40000000000000)*((1183480443*3^(1/2))/80000000000000000 + (21*3^(1/2)*((3*3^(1/2))/20 - 1/10))/3200000000000 - 16010785891/800000000000000))/(9*((9*3^(1/2))/50000000000000 - 93/200000000000000)^2), 	(20*((27009*3^(1/2))/1000000000 - 3489/50000000)*((2404758213*3^(1/2))/16000000000000000 - (21*3^(1/2)*((3*3^(1/2))/20 - 1/10))/320000000000 + 7131903/64000000000000))/(9*((9*3^(1/2))/50000000000000 - 93/200000000000000)) - ((114343521*3^(1/2))/1600000000000000 + (9943777*3^(1/2)*((3*3^(1/2))/20 - 1/10))/20000000000000 + 268316551/800000000000000)/(200*((3*3^(1/2))/100000000 - 31/400000000)) - (100*((3*3^(1/2))/10000 - 11/20000)*((3465639*3^(1/2))/1600000000000000 + (3*3^(1/2)*((3*3^(1/2))/20 - 1/10))/2000000000 - 55575441/160000000000000))/(9*((3*3^(1/2))/100000000 - 31/400000000)) + (((3*3^(1/2))/5000000 - 31/20000000)*((1665944541*3^(1/2))/32000000000000000 + (3831*3^(1/2)*((3*3^(1/2))/20 - 1/10))/200000000000000 - 160128933757/8000000000000000))/(200*((3*3^(1/2))/100000000 - 31/400000000)^2) - (20*((9*3^(1/2))/25000000 - 213/200000000)*((1183480443*3^(1/2))/80000000000000000 + (21*3^(1/2)*((3*3^(1/2))/20 - 1/10))/3200000000000 - 16010785891/800000000000000))/(9*((9*3^(1/2))/50000000000000 - 93/200000000000000)) - (100*((3*3^(1/2))/500 - 31/2000)*((5185251*3^(1/2))/16000000000000000 + 31944083711/1600000000000000))/(9*((3*3^(1/2))/100000000 - 31/400000000)) + (100*((3*3^(1/2))/10000 - 11/20000)*((3*3^(1/2))/5000000 - 31/20000000)*((5185251*3^(1/2))/16000000000000000 + 31944083711/1600000000000000))/(9*((3*3^(1/2))/100000000 - 31/400000000)^2) + (20*((9*3^(1/2))/1250000000000 - 93/5000000000000)*((27009*3^(1/2))/1000000000 - 3489/50000000)*((1183480443*3^(1/2))/80000000000000000 + (21*3^(1/2)*((3*3^(1/2))/20 - 1/10))/3200000000000 - 16010785891/800000000000000))/(9*((9*3^(1/2))/50000000000000 - 93/200000000000000)^2), 	(20201563*((3*3^(1/2))/10000 - 11/20000))/(960000000*((3*3^(1/2))/100000000 - 31/400000000)) + ((62493*3^(1/2))/16000000000 + (249937*3^(1/2)*((3*3^(1/2))/20 - 1/10))/100000000 - 23974611/32000000000)/(200*((3*3^(1/2))/100000000 - 31/400000000)) - (20*((27009*3^(1/2))/1000000000 - 3489/50000000)*((207*3^(1/2))/1280000000 + (21*3^(1/2)*((3*3^(1/2))/20 - 1/10))/32000000 + 2114643/32000000000))/(9*((9*3^(1/2))/50000000000000 - 93/200000000000000)), 	((3*3^(1/2)*((3*3^(1/2))/20 - 1/10))/8000000000 - (596441019*3^(1/2))/160000000000 + 204842381/80000000000)/(200*((3*3^(1/2))/100000000 - 31/400000000)) + (20*((27009*3^(1/2))/1000000000 - 3489/50000000)*((2107047*3^(1/2))/320000000000 - 168129/12800000000))/(9*((9*3^(1/2))/50000000000000 - 93/200000000000000)) - (100*((3*3^(1/2))/10000 - 11/20000)*((7765251*3^(1/2))/320000000000 + 5703/40000000))/(9*((3*3^(1/2))/100000000 - 31/400000000)), 	(100*((416349*3^(1/2))/320000000000 - 123711/32000000000)*((3*3^(1/2))/10000 - 11/20000))/(9*((3*3^(1/2))/100000000 - 31/400000000)) - ((20010287*3^(1/2)*((3*3^(1/2))/20 - 1/10))/8000000000 - (119986137*3^(1/2))/320000000000 + 40005943/160000000000)/(200*((3*3^(1/2))/100000000 - 31/400000000)) - (20*((27009*3^(1/2))/1000000000 - 3489/50000000)*((1031871*3^(1/2))/1600000000000 - 121359/64000000000))/(9*((9*3^(1/2))/50000000000000 - 93/200000000000000)), 	((7589019*3^(1/2))/500000000000000 + (179409213*3^(1/2)*((3*3^(1/2))/20 - 1/10))/400000000000000 - 125998557/8000000000000000)/(200*((3*3^(1/2))/100000000 - 31/400000000)) + (100*((3*3^(1/2))/10000 - 11/20000)*((4034511*3^(1/2))/1600000000000000 + (297*3^(1/2)*((3*3^(1/2))/20 - 1/10))/400000000000 + 16684749/16000000000000000))/(9*((3*3^(1/2))/100000000 - 31/400000000)) - (20*((27009*3^(1/2))/1000000000 - 3489/50000000)*((52161039*3^(1/2))/3200000000000000 + (21*3^(1/2)*((3*3^(1/2))/20 - 1/10))/32000000000000 - 117174411/8000000000000000))/(9*((9*3^(1/2))/50000000000000 - 93/200000000000000)), 	((1665944541*3^(1/2))/32000000000000000 + (3831*3^(1/2)*((3*3^(1/2))/20 - 1/10))/200000000000000 - 160128933757/8000000000000000)/(300*((3*3^(1/2))/100000000 - 31/400000000)) - ((1183480443*3^(1/2))/80000000000000000 + (21*3^(1/2)*((3*3^(1/2))/20 - 1/10))/3200000000000 - 16010785891/800000000000000)/(50000000*((9*3^(1/2))/50000000000000 - 93/200000000000000)) + ((23697*3^(1/2)*((3*3^(1/2))/20 - 1/10))/32000000000000 - (369986349*3^(1/2))/8000000000000000 + 51614439/8000000000000000)/(200*((3*3^(1/2))/100000000 - 31/400000000)) + (20*((27009*3^(1/2))/1000000000 - 3489/50000000)*((29906877*3^(1/2))/1600000000000000 + (21*3^(1/2)*((3*3^(1/2))/20 - 1/10))/32000000000000 + 5990219349/80000000000000000))/(9*((9*3^(1/2))/50000000000000 - 93/200000000000000)) - (100*((3*3^(1/2))/10000 - 11/20000)*((78898791*3^(1/2))/4000000000000000 + (21*3^(1/2)*((3*3^(1/2))/20 - 1/10))/16000000000000 + 2373464247/20000000000000000))/(9*((3*3^(1/2))/100000000 - 31/400000000)), 	(20*((27009*3^(1/2))/1000000000 - 3489/50000000)*((29900577*3^(1/2))/1600000000000000 + (21*3^(1/2)*((3*3^(1/2))/20 - 1/10))/32000000000000 + 5997450849/80000000000000000))/(9*((9*3^(1/2))/50000000000000 - 93/200000000000000)) - ((599887743*3^(1/2))/16000000000000000 - (1779879*3^(1/2)*((3*3^(1/2))/20 - 1/10))/1600000000000000 + 14540151/32000000000000000)/(200*((3*3^(1/2))/100000000 - 31/400000000)) - (100*((3*3^(1/2))/10000 - 11/20000)*((11901*3^(1/2)*((3*3^(1/2))/20 - 1/10))/32000000000000 - (4750881*3^(1/2))/2000000000000000 + 4731132549/80000000000000000))/(9*((3*3^(1/2))/100000000 - 31/400000000)) - (100*((3*3^(1/2))/20000 - 1/20000)*((1665944541*3^(1/2))/32000000000000000 + (3831*3^(1/2)*((3*3^(1/2))/20 - 1/10))/200000000000000 - 160128933757/8000000000000000))/(3*((3*3^(1/2))/100000000 - 31/400000000)) - (((11*3^(1/2))/200000000 - 3/40000000)*((1665944541*3^(1/2))/32000000000000000 + (3831*3^(1/2)*((3*3^(1/2))/20 - 1/10))/200000000000000 - 160128933757/8000000000000000))/(200*((3*3^(1/2))/100000000 - 31/400000000)^2) + (20*((99*3^(1/2))/2000000 - 27/400000)*((1183480443*3^(1/2))/80000000000000000 + (21*3^(1/2)*((3*3^(1/2))/20 - 1/10))/3200000000000 - 16010785891/800000000000000))/(9*((9*3^(1/2))/50000000000000 - 93/200000000000000)) - (100*((9*3^(1/2))/20000 - 3/20000)*((5185251*3^(1/2))/16000000000000000 + 31944083711/1600000000000000))/(9*((3*3^(1/2))/100000000 - 31/400000000)) - (100*((3*3^(1/2))/10000 - 11/20000)*((11*3^(1/2))/200000000 - 3/40000000)*((5185251*3^(1/2))/16000000000000000 + 31944083711/1600000000000000))/(9*((3*3^(1/2))/100000000 - 31/400000000)^2) - (20*((27009*3^(1/2))/1000000000 - 3489/50000000)*((33*3^(1/2))/100000000000000 - 9/20000000000000)*((1183480443*3^(1/2))/80000000000000000 + (21*3^(1/2)*((3*3^(1/2))/20 - 1/10))/3200000000000 - 16010785891/800000000000000))/(9*((9*3^(1/2))/50000000000000 - 93/200000000000000)^2), 	((891*3^(1/2))/80000000 - 417/40000000)/(200*((3*3^(1/2))/100000000 - 31/400000000)) - (20*((27009*3^(1/2))/1000000000 - 3489/50000000)*((1192731*3^(1/2))/3200000000 - 1205067/3200000000))/(9*((9*3^(1/2))/50000000000000 - 93/200000000000000)) + (100*((3*3^(1/2))/10000 - 11/20000)*((292941*3^(1/2))/800000000 - 589209/1600000000))/(9*((3*3^(1/2))/100000000 - 31/400000000)), 	((307161*3^(1/2))/800000000 - 620169/1600000000)/(200*((3*3^(1/2))/100000000 - 31/400000000)) - (20*((27009*3^(1/2))/1000000000 - 3489/50000000)*((58929*3^(1/2))/160000000 - 601209/1600000000))/(9*((9*3^(1/2))/50000000000000 - 93/200000000000000)) + (3^(1/2)*((3*3^(1/2))/10000 - 11/20000))/(20000*((3*3^(1/2))/100000000 - 31/400000000)), 	((1192731*3^(1/2))/3200000000 - 1205067/3200000000)/(200*((3*3^(1/2))/100000000 - 31/400000000)) - (100*((3*3^(1/2))/10000 - 11/20000)*((58929*3^(1/2))/160000000 - 601209/1600000000))/(9*((3*3^(1/2))/100000000 - 31/400000000)), 	0, 	0, 	0, 	0, 	0, 	0, 	0, 	0, 	0, 	0, 	0, 	0, 	1/(200*((3*3^(1/2))/100000000 - 31/400000000)), 	-(100*((3*3^(1/2))/10000 - 11/20000))/(9*((3*3^(1/2))/100000000 - 31/400000000)), 	(20*((27009*3^(1/2))/1000000000 - 3489/50000000))/(9*((9*3^(1/2))/50000000000000 - 93/200000000000000)), 	1/(200*((3*3^(1/2))/100000000 - 31/400000000)), 	-(100*((3*3^(1/2))/10000 - 11/20000))/(9*((3*3^(1/2))/100000000 - 31/400000000)), 	(20*((27009*3^(1/2))/1000000000 - 3489/50000000))/(9*((9*3^(1/2))/50000000000000 - 93/200000000000000)); 
		0, 	0, 	0, 	0, 	0, 	0, 	0, 	0, 	0, 	0, 	0, 	0, 	0, 	0, 	0, 	0, 	0, 	0, 	1, 	0, 	0, 	0, 	0, 	0, 	0, 	0, 	0, 	0, 	0, 	0, 	0, 	0, 	0, 	0, 	0, 	0; 
		0, 	0, 	0, 	0, 	0, 	0, 	0, 	0, 	0, 	0, 	0, 	0, 	0, 	0, 	0, 	0, 	0, 	0, 	0, 	1, 	0, 	0, 	0, 	0, 	0, 	0, 	0, 	0, 	0, 	0, 	0, 	0, 	0, 	0, 	0, 	0; 
		0, 	0, 	0, 	0, 	0, 	0, 	0, 	0, 	0, 	0, 	0, 	0, 	0, 	0, 	0, 	0, 	0, 	0, 	0, 	0, 	1, 	0, 	0, 	0, 	0, 	0, 	0, 	0, 	0, 	0, 	0, 	0, 	0, 	0, 	0, 	0; 
		0, 	0, 	0, 	0, 	0, 	0, 	0, 	0, 	0, 	0, 	0, 	0, 	0, 	0, 	0, 	0, 	0, 	0, 	0, 	0, 	0, 	0, 	0, 	0, 	1, 	0, 	0, 	0, 	0, 	0, 	0, 	0, 	0, 	0, 	0, 	0; 
		0, 	0, 	0, 	0, 	0, 	0, 	0, 	0, 	0, 	0, 	0, 	0, 	0, 	0, 	0, 	0, 	0, 	0, 	0, 	0, 	0, 	0, 	0, 	0, 	0, 	1, 	0, 	0, 	0, 	0, 	0, 	0, 	0, 	0, 	0, 	0; 
		0, 	0, 	0, 	0, 	0, 	0, 	0, 	0, 	0, 	0, 	0, 	0, 	0, 	0, 	0, 	0, 	0, 	0, 	0, 	0, 	0, 	0, 	0, 	0, 	0, 	0, 	1, 	0, 	0, 	0, 	0, 	0, 	0, 	0, 	0, 	0; 
		0, 	0, 	0, 	0, 	0, 	0, 	0, 	0, 	0, 	0, 	0, 	0, 	0, 	0, 	0, 	0, 	0, 	0, 	0, 	0, 	0, 	0, 	0, 	0, 	0, 	0, 	0, 	0, 	0, 	0, 	1, 	0, 	0, 	0, 	0, 	0; 
		0, 	0, 	0, 	0, 	0, 	0, 	0, 	0, 	0, 	0, 	0, 	0, 	0, 	0, 	0, 	0, 	0, 	0, 	0, 	0, 	0, 	0, 	0, 	0, 	0, 	0, 	0, 	0, 	0, 	0, 	0, 	1, 	0, 	0, 	0, 	0; 
		0, 	0, 	0, 	0, 	0, 	0, 	0, 	0, 	0, 	0, 	0, 	0, 	0, 	0, 	0, 	0, 	0, 	0, 	0, 	0, 	0, 	0, 	0, 	0, 	0, 	0, 	0, 	0, 	0, 	0, 	0, 	0, 	1, 	0, 	0, 	0];

== matlab function wrench_observer_R2016b/Subsystem/MATLAB Function1 ==
  data: eul_angl input; R_tau_e output; theta input
function R_tau_e = fcn(eul_angl,theta)
phi = eul_angl(1);
the = eul_angl(2);
psi = eul_angl(3);
theta1 = theta(1);
theta2 = theta(2);
theta3 = theta(3);
R_IB = [cos(psi)*cos(the), cos(psi)*sin(the)*sin(phi)-sin(psi)*cos(phi), cos(psi)*sin(the)*cos(phi)+sin(psi)*sin(phi);
            sin(psi)*cos(the), sin(psi)*sin(the)*sin(phi)+cos(psi)*cos(phi), sin(psi)*sin(the)*cos(phi)-cos(psi)*sin(phi);
            -sin(the), cos(the)*sin(phi), cos(the)*cos(phi)];

p_B_TCP_skew = [0, - (3*sin(theta2 + theta3))/10 - (3*sin(theta2))/10 - 1/10,(3*sin(theta1)*(cos(theta2 + theta3) + cos(theta2)))/10;
                (3*sin(theta2 + theta3))/10 + (3*sin(theta2))/10 + 1/10, 0, -(3*cos(theta1)*(cos(theta2 + theta3) + cos(theta2)))/10;
                -(3*sin(theta1)*(cos(theta2 + theta3) + cos(theta2)))/10, (3*cos(theta1)*(cos(theta2 + theta3) + cos(theta2)))/10,0];
 
R_tau_e = R_IB * p_B_TCP_skew;

== matlab function wrench_observer_R2016b/Subsystem/MATLAB Function2 ==
  data: eul_angl input; R_f_e output; theta input
function R_f_e = fcn(eul_angl,theta)
phi = eul_angl(1);
the = eul_angl(2);
psi = eul_angl(3);
theta1 = theta(1);
theta2 = theta(2);
theta3 = theta(3);
R_IB = [cos(psi)*cos(the), cos(psi)*sin(the)*sin(phi)-sin(psi)*cos(phi), cos(psi)*sin(the)*cos(phi)+sin(psi)*sin(phi);
        sin(psi)*cos(the), sin(psi)*sin(the)*sin(phi)+cos(psi)*cos(phi), sin(psi)*sin(the)*cos(phi)-cos(psi)*sin(phi);
        -sin(the), cos(the)*sin(phi), cos(the)*cos(phi)];

R_BL3 = [cos(theta2 + theta3)*cos(theta1), -sin(theta2 + theta3)*cos(theta1),  sin(theta1);
         cos(theta2 + theta3)*sin(theta1), -sin(theta2 + theta3)*sin(theta1), -cos(theta1);
         sin(theta2 + theta3), cos(theta2 + theta3), 0];
R_f_e = R_IB * R_BL3;

== matlab function wrench_observer_R2016b/Motion Equations with Manipulator /Coriolis_Matrix/Coriolis_Matrix_simplified/MATLAB Function ==
  data: C11 input; C output; C12 input; C13 input; C21 input; C22 input; C23 input; C31 input; C32 input; C33 input
function C = Coriolis_Matrix(C11,C12,C13,C21,C22,C23,C31,C32,C33)
C = zeros(9);
C = [C11,C12,C13;C21,C22,C23;C31,C32,C33];
